simulink model "MultiSizeCells"  (Simulink 10.2)
settings: Solver=ode45  StartTime=0.0  StopTime=2  RelTol=1e-3  EnableMultiTasking=on
libraries: NeuroModelerLibrary x7
settings Model: Creator=Bakhshiev  LastModifiedBy=Bakhshiev
settings DataIOCC: LimitDataPoints=on
settings OptimizationCC: ExpressionDepthLimit=2147483647  InitFltsAndDblsToZero=on
settings DebuggingCC: SolverPrmCheckMsg=warning  StateNameClashWarn=warning
settings SFSimCC: SimUseLocalCustomCode=on
settings RTWCC: RTWUseLocalCustomCode=on
settings ConfigComp: CovExternalEMLEnable=on

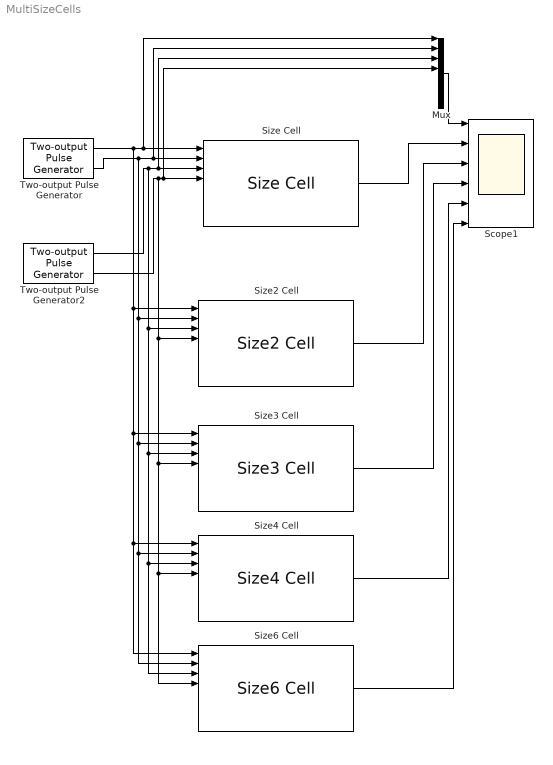
== system MultiSizeCells ==
  Mux : Mux  Inputs=8
  Scope1 : Scope  NumInputPorts=6
  Size Cell : NeuroModelerLibrary/Sized Cells/Size Cell  SystemSampleTime=-1  VariantActivationTime=update diagram  Latency=0  AutoFrameSizeCalculation=off
  Size2 Cell : NeuroModelerLibrary/Sized Cells/Size2 Cell  SystemSampleTime=-1  VariantActivationTime=update diagram  Latency=0  AutoFrameSizeCalculation=off
  Size3 Cell : NeuroModelerLibrary/Sized Cells/Size3 Cell  SystemSampleTime=-1  VariantActivationTime=update diagram  Latency=0  AutoFrameSizeCalculation=off
  Size4 Cell : NeuroModelerLibrary/Sized Cells/Size4 Cell  SystemSampleTime=-1  VariantActivationTime=update diagram  Latency=0  AutoFrameSizeCalculation=off
  Size6 Cell : NeuroModelerLibrary/Sized Cells/Size6 Cell  SystemSampleTime=-1  VariantActivationTime=update diagram  Latency=0  AutoFrameSizeCalculation=off
  Two-output Pulse Generator : NeuroModelerLibrary/Support/Two-output Pulse Generator  A=1  P1=200  P2=200  PW=1  ST=0.001  OOn1=0.5  OOff1=0.6  OOn2=0.8  OOff2=0.9
  Two-output Pulse Generator2 : NeuroModelerLibrary/Support/Two-output Pulse Generator  A=1  P1=200  P2=200  PW=1  ST=0.001  OOn1=1.2  OOff1=1.3  OOn2=1.6  OOff2=1.7
  wires:
  Two-output Pulse Generator/1 -> Mux/1, Size Cell/1, Size3 Cell/1, Size4 Cell/1, Size6 Cell/1, Size2 Cell/1
  Two-output Pulse Generator/2 -> Mux/2, Size Cell/2, Size3 Cell/2, Size4 Cell/2, Size6 Cell/2, Size2 Cell/2
  Mux/1 -> Scope1/1
  Two-output Pulse Generator2/2 -> Mux/4, Size Cell/4, Size3 Cell/4, Size4 Cell/4, Size6 Cell/4, Size2 Cell/4
  Two-output Pulse Generator2/1 -> Mux/3, Size Cell/3, Size3 Cell/3, Size4 Cell/3, Size6 Cell/3, Size2 Cell/3
  Size Cell/2 -> Scope1/2
  Size2 Cell/2 -> Scope1/3
  Size3 Cell/2 -> Scope1/4
  Size4 Cell/2 -> Scope1/5
  Size6 Cell/2 -> Scope1/6
